simulink model "FOC_PMSM"  (R2024b)
settings: Solver=ode5  StartTime=0.0  StopTime=T  FixedStep=Tsim  RelTol=1e-3
InitFcn:
  | T = 0.6;
  | Tsim = 1e-6;
  | Tcarrier = 50e-6; % fcarrier = 20kHz
  | 
  | % Treal is used to simulate
  | % real-world conditions of the MCU
  | %------------------------------
  | Treal = 25e-6;
  | 
  | % 2*Tspeed is set for the speed-loop
  | % PI controller and is slower than
  | % the current-loop PI controller
  | %--------------------------------
  | 
  | %Init:
  | % Rs = 0.62 (Ohm)
  | % Ls = 0.002075 (H)
  | % J = 36.17e-05 (kg*m^2)
  | % B = 9.444e-05 (N.m.s)
  | % K_t = 1.5*np*psi_m
  | %     = 0.51762 (N*m/A)
  |     %psi_m: flux leakage
  | % Rated currernt:
  | %   Iq = Te/Kt = 11.59A
  | 
  | np = 4;
  | ff_gain = 1;
  | 
  | %Current Loop:
  | Kp_current = 80 ;
  | Ki_current = 100 ;
  | 
  | %Speed Loop:
  | Kp_speed = 0.5;
  | Ki_speed = 30;
  | 
  | %Position Loop:
  | Kp_position = 100;
  | 
  | %====== Adaptive Fuzzy PI ========
  | um = 1;
  | em = 12;
  | D_em = 1.8;
  | 
  | kappa = 0.8;
  | epsilon = 0.01;
  | 
  | alpha = 20;
  | beta = 25;
undefined symbols (not defined in the file or in its folder): DiscIntNeverNeededParam
libraries: spsMosfetLib x12, slpidlib x8, eeTransforms x4, simulink x4, spsDCVoltageSourceLib x2, spsPermanentMagnetSynchronousMachineLib x2, SignalEditorBlockLib x2, fuzblock x1, sps_lib x1
(part 1 of 2)
settings Model: Creator=Son  LastModifiedBy=Lenovo
settings DataIOCC: ReturnWorkspaceOutputs=off
settings RTWCC: GPUComputeCapability=3.5

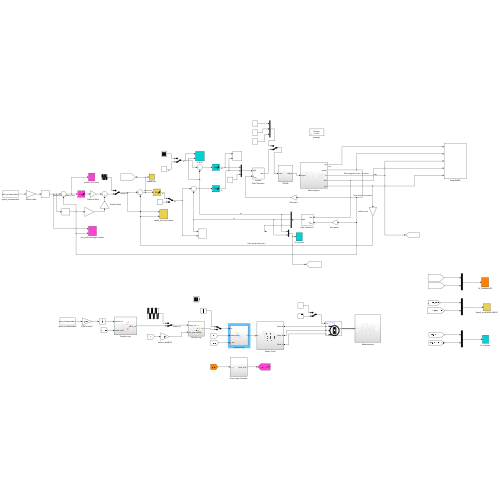
[thumbnail: Simulink's stored preview of the top-level diagram]
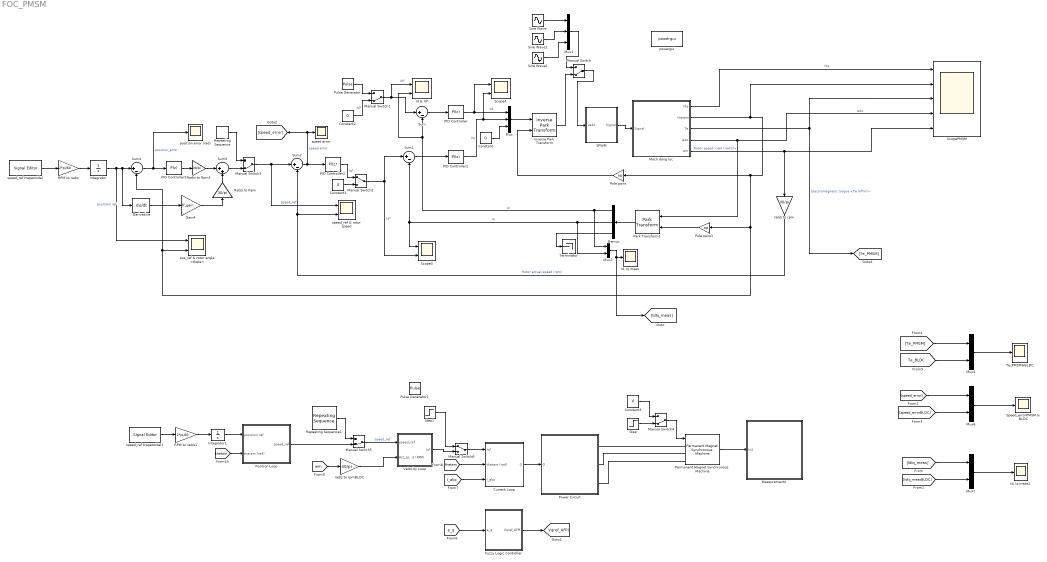
== system FOC_PMSM ==
  " Te_PMSM&BLDC" : Scope
  Constant{,1..3} (4 alike) : Constant  Value=0
  Current Loop : Subsystem
  Demux : Demux  Outputs=3
  Derivative : Derivative
  Fuzzy Logic Controller : Subsystem
  Gain4 : Gain  Gain=ff_gain
  Id & Id* : Scope  NumInputPorts=2
  "Id, Iq meas" : Scope
  "Id, Iq meas1" : Scope
  Integrator : Integrator
  Integrator1 : Integrator
  Inverse Park Transform : eeTransforms/Inverse Park Transform  AxisAlignment=D-axis  PowerInvariant=off
      settings: LibrarySourceBlock=|
      | ee_sl_lib/Mathematical
      | Transforms/Inverse
      | Park Transform
  Mach dong luc : Subsystem
  Manual Switch{,1,3..5} (5 alike) : ManualSwitch  CurrentSetting=0
  Manual Switch2 : ManualSwitch
  Manual Switch6 : ManualSwitch
  Measurements : Subsystem
  Mux : Mux  Inputs=3
  Mux1 : Mux  Inputs=3
  Mux{2,4,6..7} (4 alike) : Mux  Inputs=2
  PID Controller : slpidlib/PID Controller  Controller=PI  Form=Parallel  TimeDomain=Discrete-time  UseExternalTs=off  SampleTime=Treal  IntegratorMethod=Forward Euler  FilterMethod=Forward Euler  ControllerParametersSource=internal  P=Kp_current  I=Ki_current  UseKiTs=off  D=0  UseExternalDerivativeSource=off  N=100  UseFilter=on  TunerSelectOption=Transfer Function Based (PID Tuner App)  InitialConditionSource=internal  InitialConditionForIntegrator=0  InitialConditionForFilter=0  DifferentiatorICPrevScaledInput=0  ExternalReset=none  TrackingMode=off  Kt=1  LimitOutput=on  SatLimitsSource=internal  UpperSaturationLimit=150  LowerSaturationLimit=-150  LinearizeAsGain=on  AntiWindupMode=clamping  Kb=1  LimitIntegrator=off  UpperIntegratorSaturationLimit=inf  LowerIntegratorSaturationLimit=-inf  POutMin=[]  POutMax=[]  IOutMin=[]  IOutMax=[]  DOutMin=[]  DOutMax=[]  NOutMin=[]  NOutMax=[]  SumOutMin=[]  SumOutMax=[]  SaturationOutMin=[]  SaturationOutMax=[]  PParamMin=[]  PParamMax=[]  IParamMin=[]  IParamMax=[]  DParamMin=[]  DParamMax=[]  NParamMin=[]  NParamMax=[]  KbParamMin=[]  KbParamMax=[]  KtParamMin=[]  KtParamMax=[]  KbOutMin=[]  KbOutMax=[]  KtOutMin=[]  KtOutMax=[]  IntegratorOutMin=[]  IntegratorOutMax=[]  FilterOutMin=[]  FilterOutMax=[]  SumI1OutMin=[]  SumI1OutMax=[]  SumI2OutMin=[]  SumI2OutMax=[]  SumI3OutMin=[]  SumI3OutMax=[]  SumI4OutMin=[]  SumI4OutMax=[]  SumDOutMin=[]  SumDOutMax=[]  DifferentiatorOutMin=[]  DifferentiatorOutMax=[]  FilterDiffOutCoefMin=[]  FilterDiffOutCoefMax=[]  ReciprocalOutMin=[]  ReciprocalOutMax=[]  SumDenOutMin=[]  SumDenOutMax=[]  SumNumOutMin=[]  SumNumOutMax=[]  DivideOutMin=[]  DivideOutMax=[]  UdiffTsProdOutMin=[]  UdiffTsProdOutMax=[]  NTsProdOutMin=[]  NTsProdOutMax=[]  UintegralTsProdOutMin=[]  UintegralTsProdOutMax=[]  UngainTsProdOutMin=[]  UngainTsProdOutMax=[]  ClampingZeroOutDataTypeStr=Inherit: Inherit via back propagation  ClampingZeroOutMin=[]  ClampingZeroOutMax=[]  FilterDenConstantOutDataTypeStr=Inherit: Inherit via back propagation  FilterDenConstantOutMin=[]  FilterDenConstantOutMax=[]  PCopyOutDataTypeStr=Inherit: Inherit via back propagation  PCopyOutMin=[]  PCopyOutMax=[]  NCopyOutDataTypeStr=Inherit: Inherit via back propagation  NCopyOutMin=[]  NCopyOutMax=[]  IntegratorContinuousStateAttributes=''  IntegratorStateMustResolveToSignalObject=off  IntegratorRTWStateStorageClass=Auto  FilterContinuousStateAttributes=''  FilterStateMustResolveToSignalObject=off  FilterRTWStateStorageClass=Auto  ParallelPVariant=InternalParameters  IdealPVariant=Disabled  IVariant=InternalParameters  DVariant=Disabled  IntegratorVariant=Discrete  SatVariant=Enabled  AWVariant=DiscClampingParallel  PCopyVariant=Disabled  TRVariant=Disabled  FdbkBlocksVariant=Forward  IdealPFdbkVariant=Disabled  SatFdbkVariant=Disabled  DerivativeFilterVariant=Disabled  NVariant=Disabled  NCopyVariant=Disabled_SignalSpec  FilterICVariant=Disabled  IntegratorICVariant=InternalICs  ExternalResetVariant=Disabled  TRSumVariant=Passthrough  SumFdbkVariant=Disabled  SumVariant=Sum_PI  TsampFilterVariant=InternalTs  TsampNgainVariant=Passthrough  TsampIntegralVariant=Disabled_SignalSpec  ExternalSaturationOutDataTypeStr=Inherit: Same as second input  DerivativeSourceVariant=Disabled  PreIntVariant=InternalPreInt
  PID Controller1 : slpidlib/PID Controller  Controller=PI  Form=Parallel  TimeDomain=Discrete-time  UseExternalTs=off  SampleTime=Treal  IntegratorMethod=Forward Euler  FilterMethod=Forward Euler  ControllerParametersSource=internal  P=Kp_current  I=Ki_current  UseKiTs=off  D=0  UseExternalDerivativeSource=off  N=100  UseFilter=on  TunerSelectOption=Transfer Function Based (PID Tuner App)  InitialConditionSource=internal  InitialConditionForIntegrator=0  InitialConditionForFilter=0  DifferentiatorICPrevScaledInput=0  ExternalReset=none  TrackingMode=off  Kt=1  LimitOutput=on  SatLimitsSource=internal  UpperSaturationLimit=150  LowerSaturationLimit=-150  LinearizeAsGain=on  AntiWindupMode=clamping  Kb=1  LimitIntegrator=off  UpperIntegratorSaturationLimit=inf  LowerIntegratorSaturationLimit=-inf  POutMin=[]  POutMax=[]  IOutMin=[]  IOutMax=[]  DOutMin=[]  DOutMax=[]  NOutMin=[]  NOutMax=[]  SumOutMin=[]  SumOutMax=[]  SaturationOutMin=[]  SaturationOutMax=[]  PParamMin=[]  PParamMax=[]  IParamMin=[]  IParamMax=[]  DParamMin=[]  DParamMax=[]  NParamMin=[]  NParamMax=[]  KbParamMin=[]  KbParamMax=[]  KtParamMin=[]  KtParamMax=[]  KbOutMin=[]  KbOutMax=[]  KtOutMin=[]  KtOutMax=[]  IntegratorOutMin=[]  IntegratorOutMax=[]  FilterOutMin=[]  FilterOutMax=[]  SumI1OutMin=[]  SumI1OutMax=[]  SumI2OutMin=[]  SumI2OutMax=[]  SumI3OutMin=[]  SumI3OutMax=[]  SumI4OutMin=[]  SumI4OutMax=[]  SumDOutMin=[]  SumDOutMax=[]  DifferentiatorOutMin=[]  DifferentiatorOutMax=[]  FilterDiffOutCoefMin=[]  FilterDiffOutCoefMax=[]  ReciprocalOutMin=[]  ReciprocalOutMax=[]  SumDenOutMin=[]  SumDenOutMax=[]  SumNumOutMin=[]  SumNumOutMax=[]  DivideOutMin=[]  DivideOutMax=[]  UdiffTsProdOutMin=[]  UdiffTsProdOutMax=[]  NTsProdOutMin=[]  NTsProdOutMax=[]  UintegralTsProdOutMin=[]  UintegralTsProdOutMax=[]  UngainTsProdOutMin=[]  UngainTsProdOutMax=[]  ClampingZeroOutDataTypeStr=Inherit: Inherit via back propagation  ClampingZeroOutMin=[]  ClampingZeroOutMax=[]  FilterDenConstantOutDataTypeStr=Inherit: Inherit via back propagation  FilterDenConstantOutMin=[]  FilterDenConstantOutMax=[]  PCopyOutDataTypeStr=Inherit: Inherit via back propagation  PCopyOutMin=[]  PCopyOutMax=[]  NCopyOutDataTypeStr=Inherit: Inherit via back propagation  NCopyOutMin=[]  NCopyOutMax=[]  IntegratorContinuousStateAttributes=''  IntegratorStateMustResolveToSignalObject=off  IntegratorRTWStateStorageClass=Auto  FilterContinuousStateAttributes=''  FilterStateMustResolveToSignalObject=off  FilterRTWStateStorageClass=Auto  ParallelPVariant=InternalParameters  IdealPVariant=Disabled  IVariant=InternalParameters  DVariant=Disabled  IntegratorVariant=Discrete  SatVariant=Enabled  AWVariant=DiscClampingParallel  PCopyVariant=Disabled  TRVariant=Disabled  FdbkBlocksVariant=Forward  IdealPFdbkVariant=Disabled  SatFdbkVariant=Disabled  DerivativeFilterVariant=Disabled  NVariant=Disabled  NCopyVariant=Disabled_SignalSpec  FilterICVariant=Disabled  IntegratorICVariant=InternalICs  ExternalResetVariant=Disabled  TRSumVariant=Passthrough  SumFdbkVariant=Disabled  SumVariant=Sum_PI  TsampFilterVariant=InternalTs  TsampNgainVariant=Passthrough  TsampIntegralVariant=Disabled_SignalSpec  ExternalSaturationOutDataTypeStr=Inherit: Same as second input  DerivativeSourceVariant=Disabled  PreIntVariant=InternalPreInt
  PID Controller2 : slpidlib/PID Controller  Controller=PI  Form=Parallel  TimeDomain=Discrete-time  UseExternalTs=off  SampleTime=2*Treal  IntegratorMethod=Forward Euler  FilterMethod=Forward Euler  ControllerParametersSource=internal  P=Kp_speed  I=Ki_speed  UseKiTs=off  D=0  UseExternalDerivativeSource=off  N=100  UseFilter=on  TunerSelectOption=Transfer Function Based (PID Tuner App)  InitialConditionSource=internal  InitialConditionForIntegrator=0  InitialConditionForFilter=0  DifferentiatorICPrevScaledInput=0  ExternalReset=none  TrackingMode=off  Kt=1  LimitOutput=on  SatLimitsSource=internal  UpperSaturationLimit=11.6  LowerSaturationLimit=-11.6  LinearizeAsGain=on  AntiWindupMode=clamping  Kb=1  LimitIntegrator=off  UpperIntegratorSaturationLimit=inf  LowerIntegratorSaturationLimit=-inf  POutMin=[]  POutMax=[]  IOutMin=[]  IOutMax=[]  DOutMin=[]  DOutMax=[]  NOutMin=[]  NOutMax=[]  SumOutMin=[]  SumOutMax=[]  SaturationOutMin=[]  SaturationOutMax=[]  PParamMin=[]  PParamMax=[]  IParamMin=[]  IParamMax=[]  DParamMin=[]  DParamMax=[]  NParamMin=[]  NParamMax=[]  KbParamMin=[]  KbParamMax=[]  KtParamMin=[]  KtParamMax=[]  KbOutMin=[]  KbOutMax=[]  KtOutMin=[]  KtOutMax=[]  IntegratorOutMin=[]  IntegratorOutMax=[]  FilterOutMin=[]  FilterOutMax=[]  SumI1OutMin=[]  SumI1OutMax=[]  SumI2OutMin=[]  SumI2OutMax=[]  SumI3OutMin=[]  SumI3OutMax=[]  SumI4OutMin=[]  SumI4OutMax=[]  SumDOutMin=[]  SumDOutMax=[]  DifferentiatorOutMin=[]  DifferentiatorOutMax=[]  FilterDiffOutCoefMin=[]  FilterDiffOutCoefMax=[]  ReciprocalOutMin=[]  ReciprocalOutMax=[]  SumDenOutMin=[]  SumDenOutMax=[]  SumNumOutMin=[]  SumNumOutMax=[]  DivideOutMin=[]  DivideOutMax=[]  UdiffTsProdOutMin=[]  UdiffTsProdOutMax=[]  NTsProdOutMin=[]  NTsProdOutMax=[]  UintegralTsProdOutMin=[]  UintegralTsProdOutMax=[]  UngainTsProdOutMin=[]  UngainTsProdOutMax=[]  ClampingZeroOutDataTypeStr=Inherit: Inherit via back propagation  ClampingZeroOutMin=[]  ClampingZeroOutMax=[]  FilterDenConstantOutDataTypeStr=Inherit: Inherit via back propagation  FilterDenConstantOutMin=[]  FilterDenConstantOutMax=[]  PCopyOutDataTypeStr=Inherit: Inherit via back propagation  PCopyOutMin=[]  PCopyOutMax=[]  NCopyOutDataTypeStr=Inherit: Inherit via back propagation  NCopyOutMin=[]  NCopyOutMax=[]  IntegratorContinuousStateAttributes=''  IntegratorStateMustResolveToSignalObject=off  IntegratorRTWStateStorageClass=Auto  FilterContinuousStateAttributes=''  FilterStateMustResolveToSignalObject=off  FilterRTWStateStorageClass=Auto  ParallelPVariant=InternalParameters  IdealPVariant=Disabled  IVariant=InternalParameters  DVariant=Disabled  IntegratorVariant=Discrete  SatVariant=Enabled  AWVariant=DiscClampingParallel  PCopyVariant=Disabled  TRVariant=Disabled  FdbkBlocksVariant=Forward  IdealPFdbkVariant=Disabled  SatFdbkVariant=Disabled  DerivativeFilterVariant=Disabled  NVariant=Disabled  NCopyVariant=Disabled_SignalSpec  FilterICVariant=Disabled  IntegratorICVariant=InternalICs  ExternalResetVariant=Disabled  TRSumVariant=Passthrough  SumFdbkVariant=Disabled  SumVariant=Sum_PI  TsampFilterVariant=InternalTs  TsampNgainVariant=Passthrough  TsampIntegralVariant=Disabled_SignalSpec  ExternalSaturationOutDataTypeStr=Inherit: Same as second input  DerivativeSourceVariant=Disabled  PreIntVariant=InternalPreInt
  PID Controller3 : slpidlib/PID Controller  Controller=P  Form=Parallel  TimeDomain=Discrete-time  UseExternalTs=off  SampleTime=2*Treal  IntegratorMethod=Forward Euler  FilterMethod=Forward Euler  ControllerParametersSource=internal  P=Kp_position  I=150  UseKiTs=off  D=0  UseExternalDerivativeSource=off  N=100  UseFilter=on  TunerSelectOption=Transfer Function Based (PID Tuner App)  InitialConditionSource=internal  InitialConditionForIntegrator=0  InitialConditionForFilter=0  DifferentiatorICPrevScaledInput=0  ExternalReset=none  TrackingMode=off  Kt=1  LimitOutput=on  SatLimitsSource=internal  UpperSaturationLimit=4500  LowerSaturationLimit=-4500  LinearizeAsGain=on  AntiWindupMode=clamping  Kb=1  LimitIntegrator=off  UpperIntegratorSaturationLimit=inf  LowerIntegratorSaturationLimit=-inf  POutMin=[]  POutMax=[]  IOutMin=[]  IOutMax=[]  DOutMin=[]  DOutMax=[]  NOutMin=[]  NOutMax=[]  SumOutMin=[]  SumOutMax=[]  SaturationOutMin=[]  SaturationOutMax=[]  PParamMin=[]  PParamMax=[]  IParamMin=[]  IParamMax=[]  DParamMin=[]  DParamMax=[]  NParamMin=[]  NParamMax=[]  KbParamMin=[]  KbParamMax=[]  KtParamMin=[]  KtParamMax=[]  KbOutMin=[]  KbOutMax=[]  KtOutMin=[]  KtOutMax=[]  IntegratorOutMin=[]  IntegratorOutMax=[]  FilterOutMin=[]  FilterOutMax=[]  SumI1OutMin=[]  SumI1OutMax=[]  SumI2OutMin=[]  SumI2OutMax=[]  SumI3OutMin=[]  SumI3OutMax=[]  SumI4OutMin=[]  SumI4OutMax=[]  SumDOutMin=[]  SumDOutMax=[]  DifferentiatorOutMin=[]  DifferentiatorOutMax=[]  FilterDiffOutCoefMin=[]  FilterDiffOutCoefMax=[]  ReciprocalOutMin=[]  ReciprocalOutMax=[]  SumDenOutMin=[]  SumDenOutMax=[]  SumNumOutMin=[]  SumNumOutMax=[]  DivideOutMin=[]  DivideOutMax=[]  UdiffTsProdOutMin=[]  UdiffTsProdOutMax=[]  NTsProdOutMin=[]  NTsProdOutMax=[]  UintegralTsProdOutMin=[]  UintegralTsProdOutMax=[]  UngainTsProdOutMin=[]  UngainTsProdOutMax=[]  ClampingZeroOutDataTypeStr=Inherit: Inherit via back propagation  ClampingZeroOutMin=[]  ClampingZeroOutMax=[]  FilterDenConstantOutDataTypeStr=Inherit: Inherit via back propagation  FilterDenConstantOutMin=[]  FilterDenConstantOutMax=[]  PCopyOutDataTypeStr=Inherit: Inherit via back propagation  PCopyOutMin=[]  PCopyOutMax=[]  NCopyOutDataTypeStr=Inherit: Inherit via back propagation  NCopyOutMin=[]  NCopyOutMax=[]  IntegratorContinuousStateAttributes=''  IntegratorStateMustResolveToSignalObject=off  IntegratorRTWStateStorageClass=Auto  FilterContinuousStateAttributes=''  FilterStateMustResolveToSignalObject=off  FilterRTWStateStorageClass=Auto  ParallelPVariant=InternalParameters  IdealPVariant=Disabled  IVariant=Disabled  DVariant=Disabled  IntegratorVariant=Disabled  SatVariant=Enabled  AWVariant=Disabled  PCopyVariant=Disabled  TRVariant=Disabled  FdbkBlocksVariant=Forward  IdealPFdbkVariant=Disabled  SatFdbkVariant=Disabled  DerivativeFilterVariant=Disabled  NVariant=Disabled  NCopyVariant=Disabled_SignalSpec  FilterICVariant=Disabled  IntegratorICVariant=Disabled  ExternalResetVariant=Disabled  TRSumVariant=Passthrough  SumFdbkVariant=Disabled  SumVariant=Passthrough_P  TsampFilterVariant=InternalTs  TsampNgainVariant=Passthrough  TsampIntegralVariant=Disabled_SignalSpec  ExternalSaturationOutDataTypeStr=Inherit: Same as second input  DerivativeSourceVariant=Disabled  PreIntVariant=InternalPreInt
  Park Transform1 : eeTransforms/Park Transform  AxisAlignment=D-axis  PowerInvariant=off
      settings: LibrarySourceBlock=|
      | ee_sl_lib/Mathematical
      | Transforms/Park Transform
  Permanent Magnet Synchronous Machine : spsPermanentMagnetSynchronousMachineLib/Permanent Magnet Synchronous Machine  NbPhases=3  FluxDistribution=Trapezoidal  RotorType=Round  MechanicalLoad=Torque Tm  PresetModel="04:  6 Nm 300 Vdc 4500 RPM - 6 Nm"  ShowDetailedParameters=on  MeasurementBus=off  Resistance=0.62  Inductance=8.5e-3  dqInductances=[8.5e-3,8.5e-3]  La=0.002075  MachineConstant=Flux linkage established by magnets (V.s)  Flux=0.08627  VoltageCst=72.2734  TorqueCst=0.69016  Flat=120  Mechanical=[0.0003617 9.444e-05 4 0]  PolePairs=4  InitialConditions=[0,0, 0,0]  InitialConditions5ph=[0 0 0 0 0 0]  RefAngle=Aligned with phase A axis (original Park)  IterativeDiscreteModel=Trapezoidal non iterative  TsBlock=-1  TsPowergui=0
  Pole pairs : Gain  Gain=np
  Pole pairs1 : Gain  Gain=np
  Position Loop : Subsystem
  Power Circuit : Subsystem
  Pulse Generator : DiscretePulseGenerator  PulseType=Time based  Amplitude=6  Period=0.01  PulseWidth=50
  Pulse Generator1 : DiscretePulseGenerator  PulseType=Time based  Amplitude=50  Period=0.2  PulseWidth=50
  RPM to rad/s : Gain  Gain=2*pi/60
  RPM to rad/s1 : Gain  Gain=2*pi/60
  Rad/s to Rpm : Gain  Gain=30/pi
  Rad/s to Rpm1 : Gain  Gain=30/pi
  Repeating Sequence : simulink/Sources/Repeating Sequence  rep_seq_t=[0, 0.05, 0.08, 0.20, 0.23, 0.33, 0.36, 0.48, 0.51, 0.61]  rep_seq_y=[0, 0, 1000, 1000, 0, 0, -1000, -1000, 0, 0]
  Repeating Sequence1 : simulink/Sources/Repeating Sequence  rep_seq_t=[0, 0.05, 0.08, 0.20, 0.23, 0.33, 0.36, 0.48, 0.51, 0.61]  rep_seq_y=[0, 0, 1000, 1000, 0, 0, -1000, -1000, 0, 0]
  SPWM : Subsystem
  Scope3 : Scope  NumInputPorts=2
  Scope4 : Scope  NumInputPorts=2
  ScopePMSM : Scope  NumInputPorts=5
  Sine Wave : Sin  Amplitude=150  Frequency=2*pi*100  SampleTime=0
  Sine Wave1 : Sin  Amplitude=150  Frequency=2*pi*100  Phase=-2*pi/3  SampleTime=0
  Sine Wave2 : Sin  Amplitude=150  Frequency=2*pi*100  Phase=2*pi/3  SampleTime=0
  Speed_errorPMSM & BLDC : Scope
  Step : Step  Time=0.12  Before=0.5  After=4.5  SampleTime=0
  Step1 : Step  Time=0.1  After=11.6  SampleTime=0
  Sum{,1..2,4} (4 alike) : Sum  Inputs=|+-
  Sum5 : Sum  Inputs=|++
  Terminator : Terminator
  Velocity Loop : Subsystem
  pos_ref & rotor angle <theta> : Scope  NumInputPorts=2
  position error (rad) : Scope
  powergui : sps_lib/powergui  Priority=1  SimulationMode=Discrete  SampleTime=Tsim  frequency=60  Iterations=50  frequencyindice=0  Pbase=100e6  ErrMax=1e-4  UnitsV=kV  UnitsW=MW  buscounter=0  FunctionMessages=off  echomessages=off  EnableUseOfTLC=off  CurrentSourceSwitches=off  DisableSnubberDevices=off  DisableRonSwitches=off  DisableVfSwitches=off  DisplayEquations=off  AutomaticDiscreteSolvers=off  SolverType=Tustin/Backward Euler (TBE)  Interpol=off  ExternalGateDelay=off  methode=off  Ts=100  x0status=blocks  SPID=on  SwTol=0  HookPort=off  NonlinearTolerance=1e-4  nMaxIteration=100  ContinueOnMaxIteration=off  RestoreLinks=warning  ResistiveCurrentMeasurement=off  Frange=[0:2:500]  Ylog=off  Xlog=on  ShowGrid=off  save=off  variable=ZData  structure=0  ZoomFFT=off  StartTime=0.0  cycles=1  DisplayStyle=1  fundamental=60  FreqAxis=off  MaxFrequency=1000  frequencyindicesteady=1  RmsSteady=1  display=off
  rad/s to rpm : Gain  Gain=30/pi
  rad/s to rpmBLDC : Gain  Gain=30/pi
  speed error : Scope
  speed_ref & rotor speed : Scope  NumInputPorts=2
  speed_ref trapezoidal : SignalEditorBlockLib/Signal Editor  FileName=speed_ref_trapezoidal.mat  ActiveScenario=Scenario  ActiveSignal=speed_ref trapezoidal  IsBus=off  OutputBusObjectStr=Bus: BusObject  SampleTime=0  ZeroCross=off  OutputAfterFinalValue=Setting to zero  Unit=rpm  PreserveSignalName=on  ApplySigPropsToAllScenarios=on  ApplySigPropsToAllSignals=off
  speed_ref trapezoidal1 : SignalEditorBlockLib/Signal Editor  FileName=speed_ref_trapezoidal.mat  ActiveScenario=Scenario  ActiveSignal=speed_ref trapezoidal  IsBus=off  OutputBusObjectStr=Bus: BusObject  SampleTime=0  ZeroCross=off  OutputAfterFinalValue=Setting to zero  Unit=rpm  PreserveSignalName=on  ApplySigPropsToAllScenarios=on  ApplySigPropsToAllSignals=off
  tag scope: Vqref_AFPI=global
  wires:
  Sum1/1 -> PID Controller1/1
  Sum2/1 -> PID Controller2/1, [speed_error], speed error/1  "speed error"
  Sum/1 -> PID Controller/1
  Mach dong luc/4(Iabc) -> ScopePMSM/4, Park Transform1/1  "Iabc"
  Mach dong luc/2(thetam) -> ScopePMSM/2, Pole pairs/1, Sum4/2, pos_ref & rotor angle <theta>/2, Pole pairs1/1
  Park Transform1/1 -> Demux/1
  PID Controller3/1 -> Rad/s to Rpm1/1
  Sine Wave1/1 -> Mux1/2
  Constant/1 -> Mux/3
  Pulse Generator/1 -> Manual Switch1/1
  SPWM/1(Signal) -> Mach dong luc/1(Signal)
  Sum4/1 -> PID Controller3/1, position error (rad)/1  "position_error"
  Demux/3 -> Terminator/1
  PID Controller/1 -> Scope4/1, Mux/1  "Vd"
  Integrator/1 -> Sum4/1, Derivative/1, pos_ref & rotor angle <theta>/1  "positioin ref"
  Mach dong luc/5(wm) -> ScopePMSM/5, rad/s to rpm/1  "Rotor speed <wm (rad/s)>"
  Gain4/1 -> Rad/s to Rpm/1
  PID Controller1/1 -> Scope4/2, Mux/2  "Vq"
  Sine Wave2/1 -> Mux1/3
  RPM to rad/s/1 -> Integrator/1
  Sum5/1 -> Manual Switch3/2
  Derivative/1 -> Gain4/1
  Rad/s to Rpm1/1 -> Sum5/1
  Rad/s to Rpm/1 -> Sum5/2
  Manual Switch1/1 -> Id & Id*/1, Sum/1  "Id*"
  Manual Switch/1 -> SPWM/1(Vabc)
  Demux/1 -> Mux2/1, Id & Id*/2, Sum/2  "Id"
  Constant1/1 -> Manual Switch2/2
  PID Controller2/1 -> Manual Switch2/1  "Iq*"
  Pole pairs1/1 -> Park Transform1/2
  Manual Switch3/1 -> speed_ref & rotor speed/1, Sum2/1  "speed_ref"
  speed_ref trapezoidal/1 -> RPM to rad/s/1
  Mach dong luc/3(Te) -> [Te_PMSM], ScopePMSM/3  "Electromagnetic torque <Te (N*m)>"
  Inverse Park Transform/1 -> Manual Switch/2
  Mux1/1 -> Manual Switch/1
  Constant2/1 -> Manual Switch1/2  "Id*"
  Mux2/1 -> [IdIq_meas], "Id, Iq meas"/1
  Mach dong luc/1(Idq) -> ScopePMSM/1  "Idq"
  Pole pairs/1 -> Inverse Park Transform/2
  Demux/2 -> Mux2/2, Sum1/2, Scope3/1  "Iq"
  Manual Switch2/1 -> Scope3/2, Sum1/1  "Iq*"
  Repeating Sequence/1 -> Manual Switch3/1
  Sine Wave/1 -> Mux1/1
  rad/s to rpm/1 -> speed_ref & rotor speed/2, Sum2/2  "Rotor actual speed (rpm)"
  Mux/1 -> Inverse Park Transform/1
  speed_ref trapezoidal1/1 -> RPM to rad/s1/1
  RPM to rad/s1/1 -> Integrator1/1
  Mux4/1 -> " Te_PMSM&BLDC"/1
  Mux6/1 -> Speed_errorPMSM & BLDC/1
  Mux7/1 -> "Id, Iq meas1"/1
  [speed_error] -> Mux6/1
  [speed_errorBLDC] -> Mux6/2
  [Te_BLDC] -> Mux4/2
  [Te_PMSM] -> Mux4/1
  [IdIq_meas] -> Mux7/1
  [IdIq_measBLDC] -> Mux7/2
  Constant3/1 -> Manual Switch4/1
  Step/1 -> Manual Switch4/2
  Manual Switch4/1 -> Permanent Magnet Synchronous Machine/1
  Current Loop/1(G) -> Power Circuit/1(G)
  Permanent Magnet Synchronous Machine/1 -> Measurements/1(In4)
  [I_abc] -> Current Loop/3(I_abc)
  [thetam] -> Current Loop/2(thetam (rad))
  [wm] -> rad/s to rpmBLDC/1
  rad/s to rpmBLDC/1 -> Velocity Loop/2(Act_speed (RPM))
  Repeating Sequence1/1 -> Manual Switch5/1
  Manual Switch5/1 -> Velocity Loop/1(speed_ref)  "speed_ref"
  Integrator1/1 -> Position Loop/1(positioin ref)
  Position Loop/1(speed_ref) -> Manual Switch5/2
  [thetam] -> Position Loop/2(thetam (rad))
  Fuzzy Logic Controller/1(Vqref_AFPI) -> [Vqref_AFPI]
  [e_q] -> Fuzzy Logic Controller/1(e_q)
  Manual Switch6/1 -> Current Loop/1(Iq*)
  Velocity Loop/1(Iq*) -> Manual Switch6/2
  Step1/1 -> Manual Switch6/1
  connections:
  Permanent Magnet Synchronous Machine/LConn1 -- Power Circuit/RConn1
  Permanent Magnet Synchronous Machine/LConn2 -- Power Circuit/RConn2
  Permanent Magnet Synchronous Machine/LConn3 -- Power Circuit/RConn3

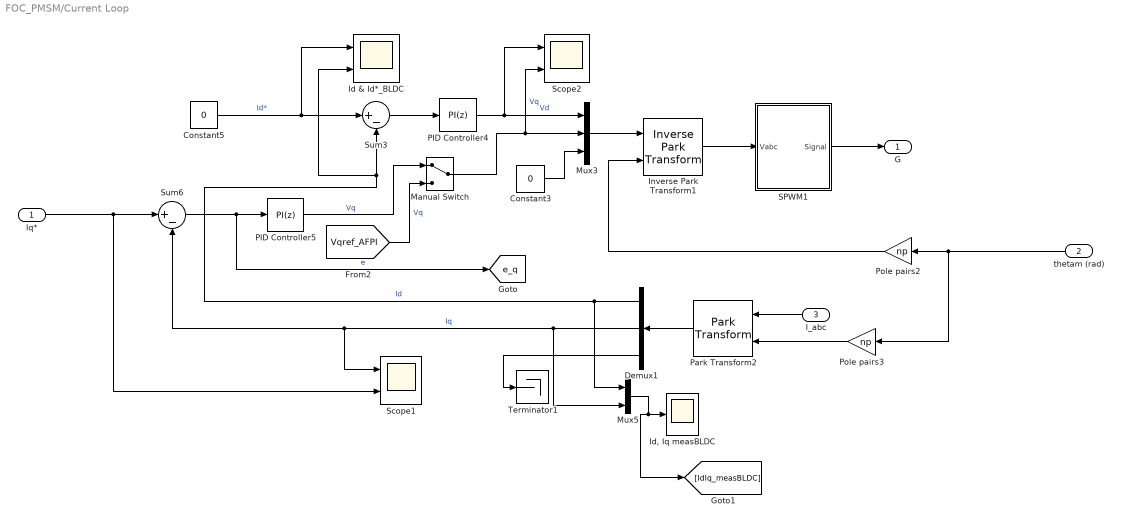
== system FOC_PMSM/Current Loop ==
  Iq* : Inport
  thetam (rad) : Inport  Port=2
  I_abc : Inport  Port=3
  Constant3 : Constant  Value=0
  Constant5 : Constant  Value=0
  Demux1 : Demux  Outputs=3
  Id & Id*_BLDC : Scope  NumInputPorts=2
  "Id, Iq measBLDC" : Scope
  Inverse Park Transform1 : eeTransforms/Inverse Park Transform  AxisAlignment=D-axis  PowerInvariant=off
      settings: LibrarySourceBlock=|
      | ee_sl_lib/Mathematical
      | Transforms/Inverse
      | Park Transform
  Manual Switch : ManualSwitch
  Mux3 : Mux  Inputs=3
  Mux5 : Mux  Inputs=2
  PID Controller4 : slpidlib/PID Controller  Controller=PI  Form=Parallel  TimeDomain=Discrete-time  UseExternalTs=off  SampleTime=Treal  IntegratorMethod=Forward Euler  FilterMethod=Forward Euler  ControllerParametersSource=internal  P=Kp_current  I=Ki_current  UseKiTs=off  D=0  UseExternalDerivativeSource=off  N=100  UseFilter=on  TunerSelectOption=Transfer Function Based (PID Tuner App)  InitialConditionSource=internal  InitialConditionForIntegrator=0  InitialConditionForFilter=0  DifferentiatorICPrevScaledInput=0  ExternalReset=none  TrackingMode=off  Kt=1  LimitOutput=on  SatLimitsSource=internal  UpperSaturationLimit=150  LowerSaturationLimit=-150  LinearizeAsGain=on  AntiWindupMode=clamping  Kb=1  LimitIntegrator=off  UpperIntegratorSaturationLimit=inf  LowerIntegratorSaturationLimit=-inf  POutMin=[]  POutMax=[]  IOutMin=[]  IOutMax=[]  DOutMin=[]  DOutMax=[]  NOutMin=[]  NOutMax=[]  SumOutMin=[]  SumOutMax=[]  SaturationOutMin=[]  SaturationOutMax=[]  PParamMin=[]  PParamMax=[]  IParamMin=[]  IParamMax=[]  DParamMin=[]  DParamMax=[]  NParamMin=[]  NParamMax=[]  KbParamMin=[]  KbParamMax=[]  KtParamMin=[]  KtParamMax=[]  KbOutMin=[]  KbOutMax=[]  KtOutMin=[]  KtOutMax=[]  IntegratorOutMin=[]  IntegratorOutMax=[]  FilterOutMin=[]  FilterOutMax=[]  SumI1OutMin=[]  SumI1OutMax=[]  SumI2OutMin=[]  SumI2OutMax=[]  SumI3OutMin=[]  SumI3OutMax=[]  SumI4OutMin=[]  SumI4OutMax=[]  SumDOutMin=[]  SumDOutMax=[]  DifferentiatorOutMin=[]  DifferentiatorOutMax=[]  FilterDiffOutCoefMin=[]  FilterDiffOutCoefMax=[]  ReciprocalOutMin=[]  ReciprocalOutMax=[]  SumDenOutMin=[]  SumDenOutMax=[]  SumNumOutMin=[]  SumNumOutMax=[]  DivideOutMin=[]  DivideOutMax=[]  UdiffTsProdOutMin=[]  UdiffTsProdOutMax=[]  NTsProdOutMin=[]  NTsProdOutMax=[]  UintegralTsProdOutMin=[]  UintegralTsProdOutMax=[]  UngainTsProdOutMin=[]  UngainTsProdOutMax=[]  ClampingZeroOutDataTypeStr=Inherit: Inherit via back propagation  ClampingZeroOutMin=[]  ClampingZeroOutMax=[]  FilterDenConstantOutDataTypeStr=Inherit: Inherit via back propagation  FilterDenConstantOutMin=[]  FilterDenConstantOutMax=[]  PCopyOutDataTypeStr=Inherit: Inherit via back propagation  PCopyOutMin=[]  PCopyOutMax=[]  NCopyOutDataTypeStr=Inherit: Inherit via back propagation  NCopyOutMin=[]  NCopyOutMax=[]  IntegratorContinuousStateAttributes=''  IntegratorStateMustResolveToSignalObject=off  IntegratorRTWStateStorageClass=Auto  FilterContinuousStateAttributes=''  FilterStateMustResolveToSignalObject=off  FilterRTWStateStorageClass=Auto  ParallelPVariant=InternalParameters  IdealPVariant=Disabled  IVariant=InternalParameters  DVariant=Disabled  IntegratorVariant=Discrete  SatVariant=Enabled  AWVariant=DiscClampingParallel  PCopyVariant=Disabled  TRVariant=Disabled  FdbkBlocksVariant=Forward  IdealPFdbkVariant=Disabled  SatFdbkVariant=Disabled  DerivativeFilterVariant=Disabled  NVariant=Disabled  NCopyVariant=Disabled_SignalSpec  FilterICVariant=Disabled  IntegratorICVariant=InternalICs  ExternalResetVariant=Disabled  TRSumVariant=Passthrough  SumFdbkVariant=Disabled  SumVariant=Sum_PI  TsampFilterVariant=InternalTs  TsampNgainVariant=Passthrough  TsampIntegralVariant=Disabled_SignalSpec  ExternalSaturationOutDataTypeStr=Inherit: Same as second input  DerivativeSourceVariant=Disabled  PreIntVariant=InternalPreInt
  PID Controller5 : slpidlib/PID Controller  Controller=PI  Form=Parallel  TimeDomain=Discrete-time  UseExternalTs=off  SampleTime=Treal  IntegratorMethod=Forward Euler  FilterMethod=Forward Euler  ControllerParametersSource=internal  P=Kp_current  I=Ki_current  UseKiTs=off  D=0  UseExternalDerivativeSource=off  N=100  UseFilter=on  TunerSelectOption=Transfer Function Based (PID Tuner App)  InitialConditionSource=internal  InitialConditionForIntegrator=0  InitialConditionForFilter=0  DifferentiatorICPrevScaledInput=0  ExternalReset=none  TrackingMode=off  Kt=1  LimitOutput=on  SatLimitsSource=internal  UpperSaturationLimit=150  LowerSaturationLimit=-150  LinearizeAsGain=on  AntiWindupMode=clamping  Kb=1  LimitIntegrator=off  UpperIntegratorSaturationLimit=inf  LowerIntegratorSaturationLimit=-inf  POutMin=[]  POutMax=[]  IOutMin=[]  IOutMax=[]  DOutMin=[]  DOutMax=[]  NOutMin=[]  NOutMax=[]  SumOutMin=[]  SumOutMax=[]  SaturationOutMin=[]  SaturationOutMax=[]  PParamMin=[]  PParamMax=[]  IParamMin=[]  IParamMax=[]  DParamMin=[]  DParamMax=[]  NParamMin=[]  NParamMax=[]  KbParamMin=[]  KbParamMax=[]  KtParamMin=[]  KtParamMax=[]  KbOutMin=[]  KbOutMax=[]  KtOutMin=[]  KtOutMax=[]  IntegratorOutMin=[]  IntegratorOutMax=[]  FilterOutMin=[]  FilterOutMax=[]  SumI1OutMin=[]  SumI1OutMax=[]  SumI2OutMin=[]  SumI2OutMax=[]  SumI3OutMin=[]  SumI3OutMax=[]  SumI4OutMin=[]  SumI4OutMax=[]  SumDOutMin=[]  SumDOutMax=[]  DifferentiatorOutMin=[]  DifferentiatorOutMax=[]  FilterDiffOutCoefMin=[]  FilterDiffOutCoefMax=[]  ReciprocalOutMin=[]  ReciprocalOutMax=[]  SumDenOutMin=[]  SumDenOutMax=[]  SumNumOutMin=[]  SumNumOutMax=[]  DivideOutMin=[]  DivideOutMax=[]  UdiffTsProdOutMin=[]  UdiffTsProdOutMax=[]  NTsProdOutMin=[]  NTsProdOutMax=[]  UintegralTsProdOutMin=[]  UintegralTsProdOutMax=[]  UngainTsProdOutMin=[]  UngainTsProdOutMax=[]  ClampingZeroOutDataTypeStr=Inherit: Inherit via back propagation  ClampingZeroOutMin=[]  ClampingZeroOutMax=[]  FilterDenConstantOutDataTypeStr=Inherit: Inherit via back propagation  FilterDenConstantOutMin=[]  FilterDenConstantOutMax=[]  PCopyOutDataTypeStr=Inherit: Inherit via back propagation  PCopyOutMin=[]  PCopyOutMax=[]  NCopyOutDataTypeStr=Inherit: Inherit via back propagation  NCopyOutMin=[]  NCopyOutMax=[]  IntegratorContinuousStateAttributes=''  IntegratorStateMustResolveToSignalObject=off  IntegratorRTWStateStorageClass=Auto  FilterContinuousStateAttributes=''  FilterStateMustResolveToSignalObject=off  FilterRTWStateStorageClass=Auto  ParallelPVariant=InternalParameters  IdealPVariant=Disabled  IVariant=InternalParameters  DVariant=Disabled  IntegratorVariant=Discrete  SatVariant=Enabled  AWVariant=DiscClampingParallel  PCopyVariant=Disabled  TRVariant=Disabled  FdbkBlocksVariant=Forward  IdealPFdbkVariant=Disabled  SatFdbkVariant=Disabled  DerivativeFilterVariant=Disabled  NVariant=Disabled  NCopyVariant=Disabled_SignalSpec  FilterICVariant=Disabled  IntegratorICVariant=InternalICs  ExternalResetVariant=Disabled  TRSumVariant=Passthrough  SumFdbkVariant=Disabled  SumVariant=Sum_PI  TsampFilterVariant=InternalTs  TsampNgainVariant=Passthrough  TsampIntegralVariant=Disabled_SignalSpec  ExternalSaturationOutDataTypeStr=Inherit: Same as second input  DerivativeSourceVariant=Disabled  PreIntVariant=InternalPreInt
  Park Transform2 : eeTransforms/Park Transform  AxisAlignment=D-axis  PowerInvariant=off
      settings: LibrarySourceBlock=|
      | ee_sl_lib/Mathematical
      | Transforms/Park Transform
  Pole pairs2 : Gain  Gain=np
  Pole pairs3 : Gain  Gain=np
  SPWM1 : Subsystem
  Scope1 : Scope  NumInputPorts=2
  Scope2 : Scope  NumInputPorts=2
  Sum3 : Sum  Inputs=|+-
  Sum6 : Sum  Inputs=|+-
  Terminator1 : Terminator
  G : Outport
  tag scope: e_q=global
  wires:
  Demux1/1 -> Sum3/2, Id & Id*_BLDC/2, Mux5/1  "Id"
  SPWM1/1(Signal) -> G/1
  Demux1/2 -> Scope1/1, Sum6/2, Mux5/2  "Iq"
  Inverse Park Transform1/1 -> SPWM1/1(Vabc)
  Demux1/3 -> Terminator1/1
  Sum6/1 -> [e_q], PID Controller5/1  "e"
  Pole pairs3/1 -> Park Transform2/2
  Constant3/1 -> Mux3/3
  Mux5/1 -> [IdIq_measBLDC], "Id, Iq measBLDC"/1
  Pole pairs2/1 -> Inverse Park Transform1/2
  Park Transform2/1 -> Demux1/1
  Sum3/1 -> PID Controller4/1
  Mux3/1 -> Inverse Park Transform1/1
  Iq*/1 -> Scope1/2, Sum6/1
  Constant5/1 -> Id & Id*_BLDC/1, Sum3/1  "Id*"
  PID Controller4/1 -> Mux3/1, Scope2/1  "Vd"
  thetam (rad)/1 -> Pole pairs3/1, Pole pairs2/1
  I_abc/1 -> Park Transform2/1
  PID Controller5/1 -> Manual Switch/1  "Vq"
  [Vqref_AFPI] -> Manual Switch/2  "Vq"
  Manual Switch/1 -> Scope2/2, Mux3/2  "Vq"

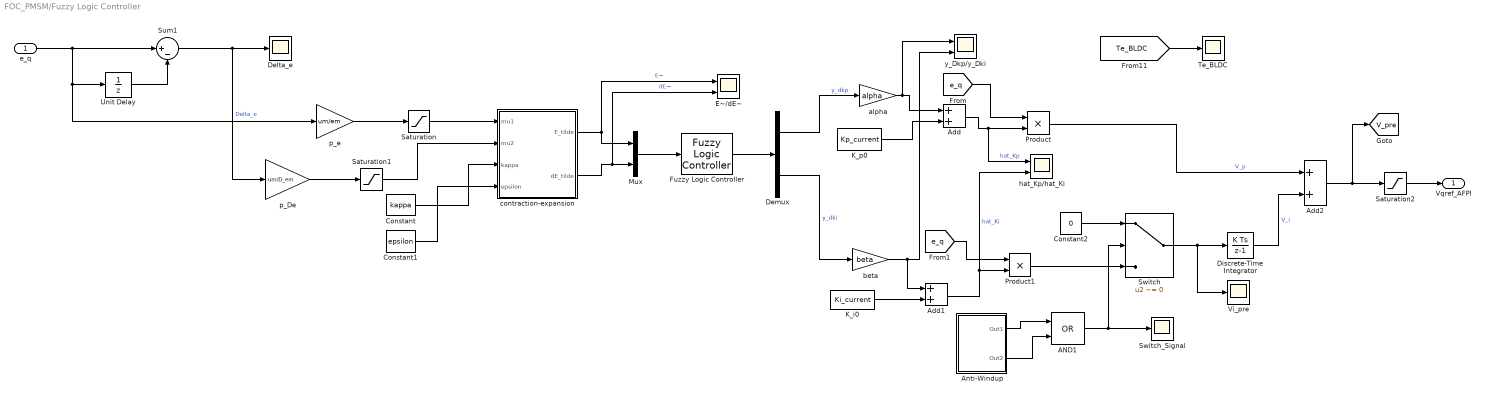
== system FOC_PMSM/Fuzzy Logic Controller ==
  e_q : Inport
  AND1 : Logic  Operator=OR  IconShape=distinctive  AllPortsSameDT=off  OutDataTypeStr=boolean
  Add : Sum
  Add1 : Sum
  Add2 : Sum
  Anti-Windup : Subsystem
  Constant : Constant  Value=kappa
  Constant1 : Constant  Value=epsilon
  Constant2 : Constant  Value=0
  Delta_e : Scope
  Demux : Demux  Outputs=2
  Discrete-Time Integrator : DiscreteIntegrator  SampleTime=Treal  ICPrevOutput=DiscIntNeverNeededParam  ICPrevScaledInput=DiscIntNeverNeededParam
  E~/dE~ : Scope  NumInputPorts=2
  Fuzzy Logic Controller : fuzblock/Fuzzy Logic  Controller  FIS=myFIS  OutputSampleNumber=101  DataType=double  FuzzifiedInputs=off  RuleFiringStrengths=off  RuleOutputs=off  AggregatedOutputs=off  SimulateUsing=Code generation  OutOfRangeInputValueMessage=warning  NoRuleFiredMessage=warning  EmptyOutputFuzzySetMessage=warning
  K_i0 : Constant  Value=Ki_current
  K_p0 : Constant  Value=Kp_current
  Mux : Mux  Inputs=2
  Product : Product
  Product1 : Product
  Saturation : Saturate  UpperLimit=1  LowerLimit=-1
  Saturation1 : Saturate  UpperLimit=1  LowerLimit=-1
  Saturation2 : Saturate  UpperLimit=150  LowerLimit=-150
  Sum1 : Sum  Inputs=|+-
  Switch : Switch  Criteria=u2 ~= 0  Threshold=150  SaturateOnIntegerOverflow=off  InputSameDT=off
  Switch_Signal : Scope
  Te_BLDC : Scope
  Unit Delay : UnitDelay  SampleTime=Treal  HasFrameUpgradeWarning=on
  Vi_pre : Scope
  alpha : Gain  Gain=alpha
  beta : Gain  Gain=beta
  "contraction-expansion " : MATLAB Function  TreatAsAtomicUnit=on
  hat_Kp/hat_Ki : Scope  NumInputPorts=2
  p_De : Gain  Gain=um/D_em
  p_e : Gain  Gain=um/em
  y_Dkp/y_Dki : Scope  NumInputPorts=2
  Vqref_AFPI : Outport
  tag scope: V_pre=global
  wires:
  Demux/1 -> alpha/1  "y_dkp"
  e_q/1 -> p_e/1, Unit Delay/1, Sum1/1
  Constant2/1 -> Switch/1
  beta/1 -> y_Dkp/y_Dki/2, Add1/1
  Constant1/1 -> "contraction-expansion "/4(epsilon)
  p_De/1 -> Saturation1/1
  Constant/1 -> "contraction-expansion "/3(kappa)
  alpha/1 -> y_Dkp/y_Dki/1, Add/1
  Saturation1/1 -> "contraction-expansion "/2(mu2)
  K_p0/1 -> Add/2
  Sum1/1 -> p_De/1, Delta_e/1  "Delta_e"
  Product1/1 -> Switch/3
  Demux/2 -> beta/1  "y_dki"
  K_i0/1 -> Add1/2
  [e_q] -> Product1/1
  Add2/1 -> [V_pre], Saturation2/1
  Product/1 -> Add2/1  "V_p"
  Unit Delay/1 -> Sum1/2
  Saturation2/1 -> Vqref_AFPI/1
  Fuzzy Logic Controller/1 -> Demux/1
  "contraction-expansion "/1(E_tilde) -> E~/dE~/1, Mux/1  "E~"
  Saturation/1 -> "contraction-expansion "/1(mu1)
  Switch/1 -> Vi_pre/1, Discrete-Time Integrator/1
  Add1/1 -> hat_Kp/hat_Ki/2, Product1/2  "hat_Ki"
  Discrete-Time Integrator/1 -> Add2/2  "V_i"
  p_e/1 -> Saturation/1
  Add/1 -> hat_Kp/hat_Ki/1, Product/2  "hat_Kp"
  [e_q] -> Product/1
  Mux/1 -> Fuzzy Logic Controller/1
  "contraction-expansion "/2(dE_tilde) -> E~/dE~/2, Mux/2  "dE~"
  Anti-Windup/1(Out1) -> AND1/1
  Anti-Windup/2(Out2) -> AND1/2
  AND1/1 -> Switch/2, Switch_Signal/1
  [Te_BLDC] -> Te_BLDC/1

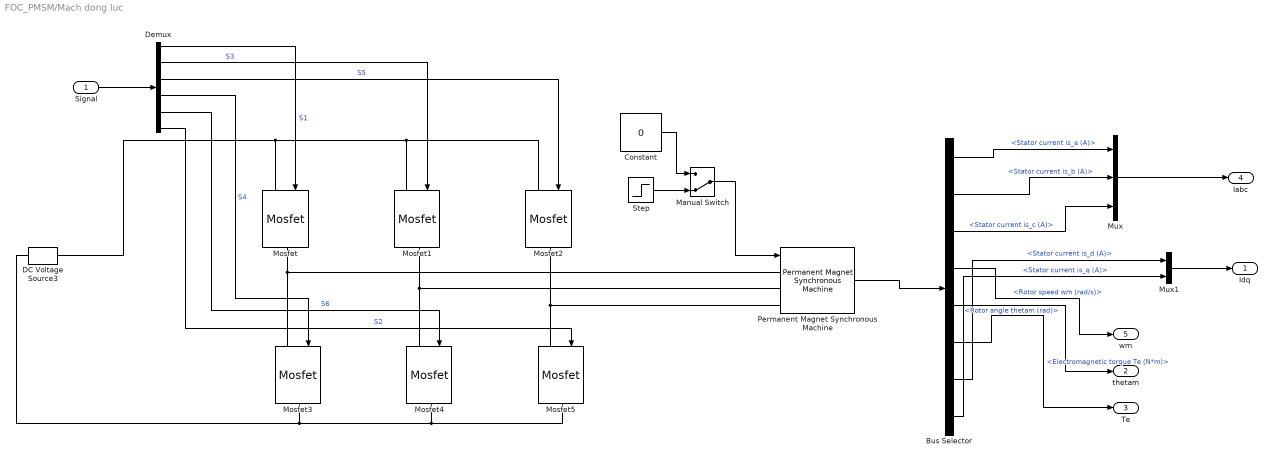
== system FOC_PMSM/Mach dong luc ==
  Signal : Inport
  Bus Selector : BusSelector  OutputSignals=Stator current is_a (A),Stator current is_b (A),Stator current is_c (A),Rotor speed wm (rad/s),Rotor angle thetam (rad),Electromagnetic torque Te (N*m),Stator current is_d (A),Stator current is_q (A)
  Constant : Constant  Value=0
  DC Voltage Source3 : spsDCVoltageSourceLib/DC Voltage Source  Amplitude=300  Measurements=None
  Demux : Demux  Outputs=6
  Manual Switch : ManualSwitch  CurrentSetting=0
  Mosfet{,1..5} (6 alike) : spsMosfetLib/Mosfet  Ron=0.1  Lon=0  Rd=0.01  Vfd=0  IC=0  Rs=1e5  Cs=inf  Measurements=off
  Mux : Mux  Inputs=3
  Mux1 : Mux  Inputs=2
  Permanent Magnet Synchronous Machine : spsPermanentMagnetSynchronousMachineLib/Permanent Magnet Synchronous Machine  NbPhases=3  FluxDistribution=Sinusoidal  RotorType=Round  MechanicalLoad=Torque Tm  PresetModel="04:  6 Nm 300 Vdc 4500 RPM - 6 Nm"  ShowDetailedParameters=on  MeasurementBus=off  Resistance=0.62  Inductance=8.5e-3  dqInductances=[8.5e-3,8.5e-3]  La=0.002075  MachineConstant=Flux linkage established by magnets (V.s)  Flux=0.08627  VoltageCst=62.5906  TorqueCst=0.51762  Flat=120  Mechanical=[0.0003617 9.444e-05 4 0]  PolePairs=4  InitialConditions=[0,0, 0,0]  InitialConditions5ph=[0 0 0 0 0 0]  RefAngle=Aligned with phase A axis (original Park)  IterativeDiscreteModel=Trapezoidal non iterative  TsBlock=-1  TsPowergui=0
  Step : Step  Time=0.12  Before=0.5  After=4.5  SampleTime=0
  Idq : Outport
  thetam : Outport  Port=2
  Te : Outport  Port=3
  Iabc : Outport  Port=4
  wm : Outport  Port=5
  wires:
  Signal/1 -> Demux/1
  Demux/1 -> Mosfet/1  "S1"
  Demux/2 -> Mosfet1/1  "S3"
  Demux/3 -> Mosfet2/1  "S5"
  Demux/4 -> Mosfet3/1  "S4"
  Demux/5 -> Mosfet4/1  "S6"
  Demux/6 -> Mosfet5/1  "S2"
  Permanent Magnet Synchronous Machine/1 -> Bus Selector/1
  Bus Selector/1 -> Mux/1  "<Stator current is_a (A)>"
  Bus Selector/2 -> Mux/2  "<Stator current is_b (A)>"
  Bus Selector/3 -> Mux/3  "<Stator current is_c (A)>"
  Bus Selector/4 -> wm/1  "<Rotor speed wm (rad/s)>"
  Bus Selector/5 -> thetam/1  "<Rotor angle thetam (rad)>"
  Bus Selector/6 -> Te/1  "<Electromagnetic torque Te (N*m)>"
  Mux/1 -> Iabc/1
  Mux1/1 -> Idq/1
  Manual Switch/1 -> Permanent Magnet Synchronous Machine/1
  Step/1 -> Manual Switch/2
  Constant/1 -> Manual Switch/1
  Bus Selector/7 -> Mux1/1  "<Stator current is_d (A)>"
  Bus Selector/8 -> Mux1/2  "<Stator current is_q (A)>"
  connections:
  Permanent Magnet Synchronous Machine/LConn1 -- Mosfet/RConn1 -- Mosfet3/LConn1
  Permanent Magnet Synchronous Machine/LConn2 -- Mosfet1/RConn1 -- Mosfet4/LConn1
  Permanent Magnet Synchronous Machine/LConn3 -- Mosfet2/RConn1 -- Mosfet5/LConn1
  Mosfet5/RConn1 -- Mosfet4/RConn1 -- DC Voltage Source3/LConn1 -- Mosfet3/RConn1
  Mosfet/LConn1 -- DC Voltage Source3/RConn1 -- Mosfet2/LConn1 -- Mosfet1/LConn1

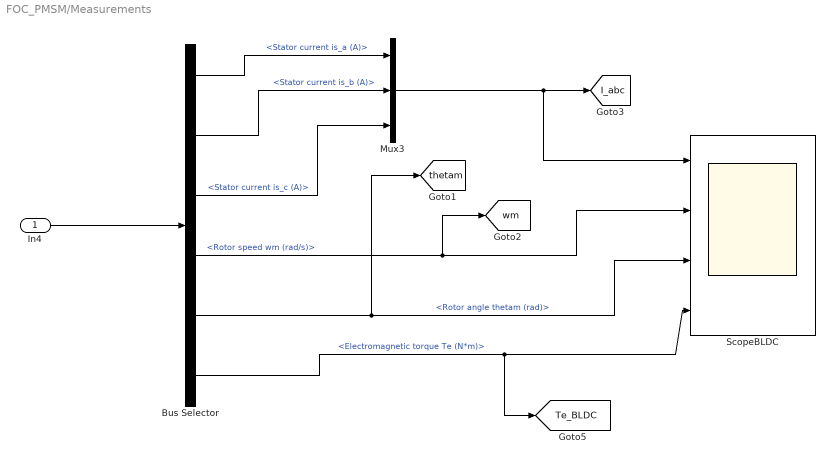
== system FOC_PMSM/Measurements ==
  In4 : Inport
  Bus Selector : BusSelector  OutputSignals=Stator current is_a (A),Stator current is_b (A),Stator current is_c (A),Rotor speed wm (rad/s),Rotor angle thetam (rad),Electromagnetic torque Te (N*m)
  Mux3 : Mux  Inputs=3
  ScopeBLDC : Scope  NumInputPorts=4
  tag scope: I_abc=global, Te_BLDC=global, thetam=global, wm=global
  wires:
  Mux3/1 -> [I_abc], ScopeBLDC/1
  Bus Selector/2 -> Mux3/2  "<Stator current is_b (A)>"
  In4/1 -> Bus Selector/1
  Bus Selector/3 -> Mux3/3  "<Stator current is_c (A)>"
  Bus Selector/1 -> Mux3/1  "<Stator current is_a (A)>"
  Bus Selector/5 -> [thetam], ScopeBLDC/3  "<Rotor angle thetam (rad)>"
  Bus Selector/4 -> [wm], ScopeBLDC/2  "<Rotor speed wm (rad/s)>"
  Bus Selector/6 -> [Te_BLDC], ScopeBLDC/4  "<Electromagnetic torque Te (N*m)>"

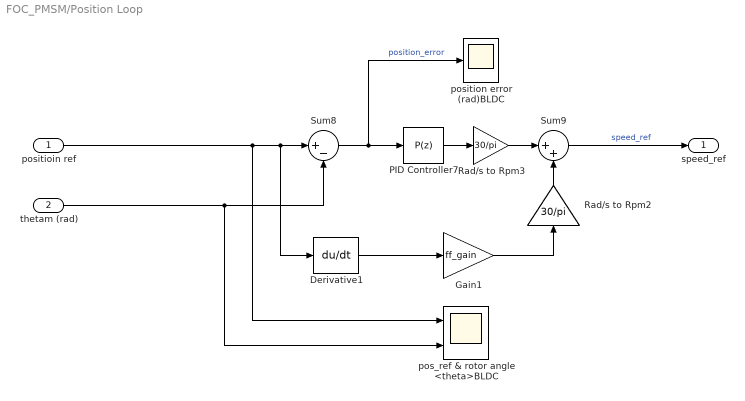
== system FOC_PMSM/Position Loop ==
  positioin ref : Inport
  thetam (rad) : Inport  Port=2
  Derivative1 : Derivative
  Gain1 : Gain  Gain=ff_gain
  PID Controller7 : slpidlib/PID Controller  Controller=P  Form=Parallel  TimeDomain=Discrete-time  UseExternalTs=off  SampleTime=2*Treal  IntegratorMethod=Forward Euler  FilterMethod=Forward Euler  ControllerParametersSource=internal  P=Kp_position  I=150  UseKiTs=off  D=0  UseExternalDerivativeSource=off  N=100  UseFilter=on  TunerSelectOption=Transfer Function Based (PID Tuner App)  InitialConditionSource=internal  InitialConditionForIntegrator=0  InitialConditionForFilter=0  DifferentiatorICPrevScaledInput=0  ExternalReset=none  TrackingMode=off  Kt=1  LimitOutput=on  SatLimitsSource=internal  UpperSaturationLimit=4500  LowerSaturationLimit=-4500  LinearizeAsGain=on  AntiWindupMode=clamping  Kb=1  LimitIntegrator=off  UpperIntegratorSaturationLimit=inf  LowerIntegratorSaturationLimit=-inf  POutMin=[]  POutMax=[]  IOutMin=[]  IOutMax=[]  DOutMin=[]  DOutMax=[]  NOutMin=[]  NOutMax=[]  SumOutMin=[]  SumOutMax=[]  SaturationOutMin=[]  SaturationOutMax=[]  PParamMin=[]  PParamMax=[]  IParamMin=[]  IParamMax=[]  DParamMin=[]  DParamMax=[]  NParamMin=[]  NParamMax=[]  KbParamMin=[]  KbParamMax=[]  KtParamMin=[]  KtParamMax=[]  KbOutMin=[]  KbOutMax=[]  KtOutMin=[]  KtOutMax=[]  IntegratorOutMin=[]  IntegratorOutMax=[]  FilterOutMin=[]  FilterOutMax=[]  SumI1OutMin=[]  SumI1OutMax=[]  SumI2OutMin=[]  SumI2OutMax=[]  SumI3OutMin=[]  SumI3OutMax=[]  SumI4OutMin=[]  SumI4OutMax=[]  SumDOutMin=[]  SumDOutMax=[]  DifferentiatorOutMin=[]  DifferentiatorOutMax=[]  FilterDiffOutCoefMin=[]  FilterDiffOutCoefMax=[]  ReciprocalOutMin=[]  ReciprocalOutMax=[]  SumDenOutMin=[]  SumDenOutMax=[]  SumNumOutMin=[]  SumNumOutMax=[]  DivideOutMin=[]  DivideOutMax=[]  UdiffTsProdOutMin=[]  UdiffTsProdOutMax=[]  NTsProdOutMin=[]  NTsProdOutMax=[]  UintegralTsProdOutMin=[]  UintegralTsProdOutMax=[]  UngainTsProdOutMin=[]  UngainTsProdOutMax=[]  ClampingZeroOutDataTypeStr=Inherit: Inherit via back propagation  ClampingZeroOutMin=[]  ClampingZeroOutMax=[]  FilterDenConstantOutDataTypeStr=Inherit: Inherit via back propagation  FilterDenConstantOutMin=[]  FilterDenConstantOutMax=[]  PCopyOutDataTypeStr=Inherit: Inherit via back propagation  PCopyOutMin=[]  PCopyOutMax=[]  NCopyOutDataTypeStr=Inherit: Inherit via back propagation  NCopyOutMin=[]  NCopyOutMax=[]  IntegratorContinuousStateAttributes=''  IntegratorStateMustResolveToSignalObject=off  IntegratorRTWStateStorageClass=Auto  FilterContinuousStateAttributes=''  FilterStateMustResolveToSignalObject=off  FilterRTWStateStorageClass=Auto  ParallelPVariant=InternalParameters  IdealPVariant=Disabled  IVariant=Disabled  DVariant=Disabled  IntegratorVariant=Disabled  SatVariant=Enabled  AWVariant=Disabled  PCopyVariant=Disabled  TRVariant=Disabled  FdbkBlocksVariant=Forward  IdealPFdbkVariant=Disabled  SatFdbkVariant=Disabled  DerivativeFilterVariant=Disabled  NVariant=Disabled  NCopyVariant=Disabled_SignalSpec  FilterICVariant=Disabled  IntegratorICVariant=Disabled  ExternalResetVariant=Disabled  TRSumVariant=Passthrough  SumFdbkVariant=Disabled  SumVariant=Passthrough_P  TsampFilterVariant=InternalTs  TsampNgainVariant=Passthrough  TsampIntegralVariant=Disabled_SignalSpec  ExternalSaturationOutDataTypeStr=Inherit: Same as second input  DerivativeSourceVariant=Disabled  PreIntVariant=InternalPreInt
  Rad/s to Rpm2 : Gain  Gain=30/pi
  Rad/s to Rpm3 : Gain  Gain=30/pi
  Sum8 : Sum  Inputs=|+-
  Sum9 : Sum  Inputs=|++
  pos_ref & rotor angle <theta>BLDC : Scope  NumInputPorts=2
  position error (rad)BLDC : Scope
  speed_ref : Outport
  wires:
  thetam (rad)/1 -> pos_ref & rotor angle <theta>BLDC/2, Sum8/2
  Sum8/1 -> position error (rad)BLDC/1, PID Controller7/1  "position_error"
  Rad/s to Rpm2/1 -> Sum9/2
  positioin ref/1 -> Sum8/1, Derivative1/1, pos_ref & rotor angle <theta>BLDC/1
  Rad/s to Rpm3/1 -> Sum9/1
  Derivative1/1 -> Gain1/1
  Gain1/1 -> Rad/s to Rpm2/1
  PID Controller7/1 -> Rad/s to Rpm3/1
  Sum9/1 -> speed_ref/1  "speed_ref"

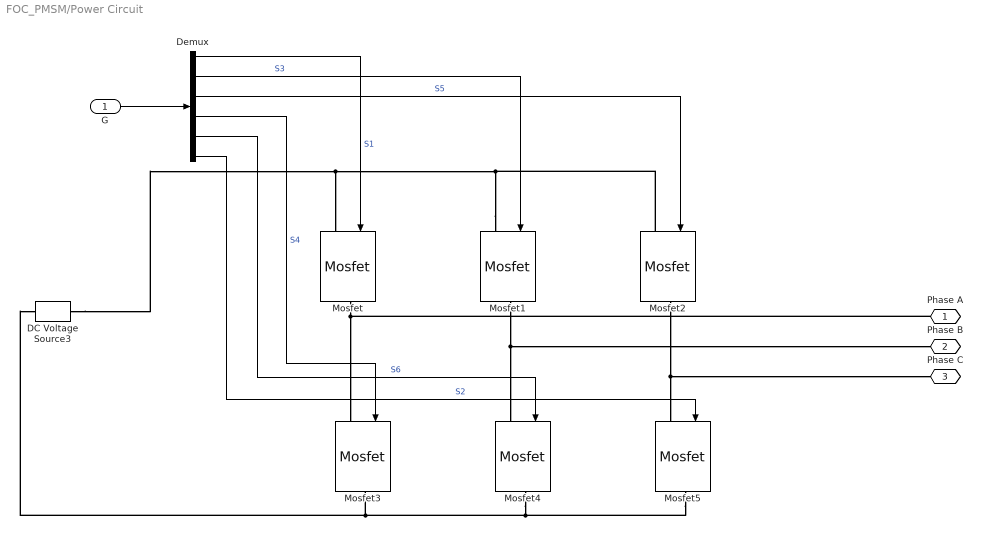
== system FOC_PMSM/Power Circuit ==
  G : Inport
  DC Voltage Source3 : spsDCVoltageSourceLib/DC Voltage Source  Amplitude=300  Measurements=None
  Demux : Demux  Outputs=6
  Mosfet{,1..5} (6 alike) : spsMosfetLib/Mosfet  Ron=0.1  Lon=0  Rd=0.01  Vfd=0  IC=0  Rs=1e5  Cs=inf  Measurements=off
  Phase A : PMIOPort  Side=Right
  Phase B : PMIOPort  Port=2  Side=Right
  Phase C : PMIOPort  Port=3  Side=Right
  wires:
  Demux/6 -> Mosfet5/1  "S2"
  Demux/5 -> Mosfet4/1  "S6"
  Demux/4 -> Mosfet3/1  "S4"
  Demux/3 -> Mosfet2/1  "S5"
  Demux/2 -> Mosfet1/1  "S3"
  Demux/1 -> Mosfet/1  "S1"
  G/1 -> Demux/1
  connections:
  Mosfet1/LConn1 -- Mosfet2/LConn1 -- DC Voltage Source3/RConn1 -- Mosfet/LConn1
  Mosfet3/RConn1 -- DC Voltage Source3/LConn1 -- Mosfet4/RConn1 -- Mosfet5/RConn1
  Mosfet2/RConn1 -- Mosfet5/LConn1 -- Phase C/RConn1
  Mosfet1/RConn1 -- Phase B/RConn1 -- Mosfet4/LConn1
  Mosfet/RConn1 -- Mosfet3/LConn1 -- Phase A/RConn1

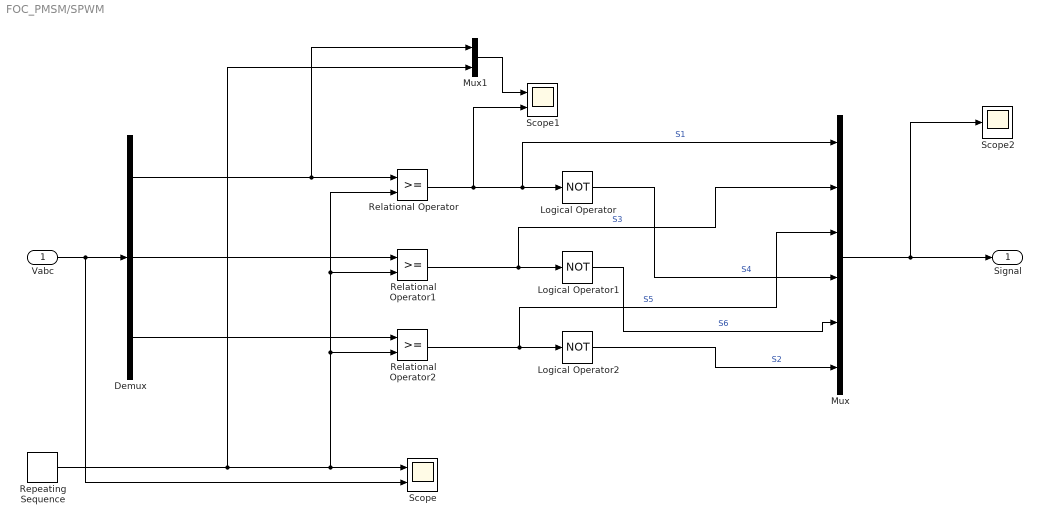
== system FOC_PMSM/SPWM ==
  Vabc : Inport
  Demux : Demux  Outputs=3
  Logical Operator : Logic  Operator=NOT  AllPortsSameDT=off  OutDataTypeStr=boolean
  Logical Operator1 : Logic  Operator=NOT  AllPortsSameDT=off  OutDataTypeStr=boolean
  Logical Operator2 : Logic  Operator=NOT  AllPortsSameDT=off  OutDataTypeStr=boolean
  Mux : Mux  Inputs=6
  Mux1 : Mux  Inputs=2
  Relational Operator : RelationalOperator  OutDataTypeStr=boolean  RndMeth=Simplest  InputSameDT=off
  Relational Operator1 : RelationalOperator  OutDataTypeStr=boolean  RndMeth=Simplest  InputSameDT=off
  Relational Operator2 : RelationalOperator  OutDataTypeStr=boolean  RndMeth=Simplest  InputSameDT=off
  Repeating Sequence : simulink/Sources/Repeating Sequence  rep_seq_t=[0, 0.5*Tcarrier, Tcarrier]  rep_seq_y=[-150, 150, -150]
  Scope : Scope  NumInputPorts=2
  Scope1 : Scope  NumInputPorts=2
  Scope2 : Scope
  Signal : Outport
  wires:
  Vabc/1 -> Scope/2, Demux/1
  Demux/1 -> Mux1/1, Relational Operator/1
  Repeating Sequence/1 -> Mux1/2, Relational Operator/2, Relational Operator1/2, Relational Operator2/2, Scope/1
  Demux/2 -> Relational Operator1/1
  Demux/3 -> Relational Operator2/1
  Relational Operator/1 -> Scope1/2, Mux/1, Logical Operator/1  "S1"
  Relational Operator1/1 -> Mux/2, Logical Operator1/1  "S3"
  Relational Operator2/1 -> Mux/3, Logical Operator2/1  "S5"
  Logical Operator/1 -> Mux/4  "S4"
  Logical Operator1/1 -> Mux/5  "S6"
  Logical Operator2/1 -> Mux/6  "S2"
  Mux/1 -> Scope2/1, Signal/1
  Mux1/1 -> Scope1/1

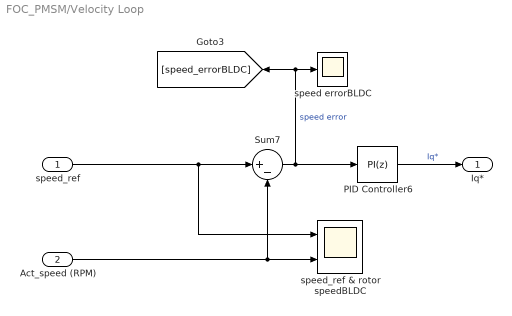
== system FOC_PMSM/Velocity Loop ==
  speed_ref : Inport
  Act_speed (RPM) : Inport  Port=2
  PID Controller6 : slpidlib/PID Controller  Controller=PI  Form=Parallel  TimeDomain=Discrete-time  UseExternalTs=off  SampleTime=2*Treal  IntegratorMethod=Forward Euler  FilterMethod=Forward Euler  ControllerParametersSource=internal  P=Kp_speed  I=Ki_speed  UseKiTs=off  D=0  UseExternalDerivativeSource=off  N=100  UseFilter=on  TunerSelectOption=Transfer Function Based (PID Tuner App)  InitialConditionSource=internal  InitialConditionForIntegrator=0  InitialConditionForFilter=0  DifferentiatorICPrevScaledInput=0  ExternalReset=none  TrackingMode=off  Kt=1  LimitOutput=on  SatLimitsSource=internal  UpperSaturationLimit=11.6  LowerSaturationLimit=-11.6  LinearizeAsGain=on  AntiWindupMode=clamping  Kb=1  LimitIntegrator=off  UpperIntegratorSaturationLimit=inf  LowerIntegratorSaturationLimit=-inf  POutMin=[]  POutMax=[]  IOutMin=[]  IOutMax=[]  DOutMin=[]  DOutMax=[]  NOutMin=[]  NOutMax=[]  SumOutMin=[]  SumOutMax=[]  SaturationOutMin=[]  SaturationOutMax=[]  PParamMin=[]  PParamMax=[]  IParamMin=[]  IParamMax=[]  DParamMin=[]  DParamMax=[]  NParamMin=[]  NParamMax=[]  KbParamMin=[]  KbParamMax=[]  KtParamMin=[]  KtParamMax=[]  KbOutMin=[]  KbOutMax=[]  KtOutMin=[]  KtOutMax=[]  IntegratorOutMin=[]  IntegratorOutMax=[]  FilterOutMin=[]  FilterOutMax=[]  SumI1OutMin=[]  SumI1OutMax=[]  SumI2OutMin=[]  SumI2OutMax=[]  SumI3OutMin=[]  SumI3OutMax=[]  SumI4OutMin=[]  SumI4OutMax=[]  SumDOutMin=[]  SumDOutMax=[]  DifferentiatorOutMin=[]  DifferentiatorOutMax=[]  FilterDiffOutCoefMin=[]  FilterDiffOutCoefMax=[]  ReciprocalOutMin=[]  ReciprocalOutMax=[]  SumDenOutMin=[]  SumDenOutMax=[]  SumNumOutMin=[]  SumNumOutMax=[]  DivideOutMin=[]  DivideOutMax=[]  UdiffTsProdOutMin=[]  UdiffTsProdOutMax=[]  NTsProdOutMin=[]  NTsProdOutMax=[]  UintegralTsProdOutMin=[]  UintegralTsProdOutMax=[]  UngainTsProdOutMin=[]  UngainTsProdOutMax=[]  ClampingZeroOutDataTypeStr=Inherit: Inherit via back propagation  ClampingZeroOutMin=[]  ClampingZeroOutMax=[]  FilterDenConstantOutDataTypeStr=Inherit: Inherit via back propagation  FilterDenConstantOutMin=[]  FilterDenConstantOutMax=[]  PCopyOutDataTypeStr=Inherit: Inherit via back propagation  PCopyOutMin=[]  PCopyOutMax=[]  NCopyOutDataTypeStr=Inherit: Inherit via back propagation  NCopyOutMin=[]  NCopyOutMax=[]  IntegratorContinuousStateAttributes=''  IntegratorStateMustResolveToSignalObject=off  IntegratorRTWStateStorageClass=Auto  FilterContinuousStateAttributes=''  FilterStateMustResolveToSignalObject=off  FilterRTWStateStorageClass=Auto  ParallelPVariant=InternalParameters  IdealPVariant=Disabled  IVariant=InternalParameters  DVariant=Disabled  IntegratorVariant=Discrete  SatVariant=Enabled  AWVariant=DiscClampingParallel  PCopyVariant=Disabled  TRVariant=Disabled  FdbkBlocksVariant=Forward  IdealPFdbkVariant=Disabled  SatFdbkVariant=Disabled  DerivativeFilterVariant=Disabled  NVariant=Disabled  NCopyVariant=Disabled_SignalSpec  FilterICVariant=Disabled  IntegratorICVariant=InternalICs  ExternalResetVariant=Disabled  TRSumVariant=Passthrough  SumFdbkVariant=Disabled  SumVariant=Sum_PI  TsampFilterVariant=InternalTs  TsampNgainVariant=Passthrough  TsampIntegralVariant=Disabled_SignalSpec  ExternalSaturationOutDataTypeStr=Inherit: Same as second input  DerivativeSourceVariant=Disabled  PreIntVariant=InternalPreInt
  Sum7 : Sum  Inputs=|+-
  speed errorBLDC : Scope
  speed_ref & rotor speedBLDC : Scope  NumInputPorts=2
  Iq* : Outport
  wires:
  Sum7/1 -> [speed_errorBLDC], speed errorBLDC/1, PID Controller6/1  "speed error"
  speed_ref/1 -> speed_ref & rotor speedBLDC/1, Sum7/1
  Act_speed (RPM)/1 -> speed_ref & rotor speedBLDC/2, Sum7/2
  PID Controller6/1 -> Iq*/1  "Iq*"
